simulink model "tm_func"  (R2026a)
settings: Solver=VariableStepAuto  StopTime=100
values from neighbouring files (symbols this model uses):
  q0 = (1 + a - 2*pd) / b    [questao6.m]
  q1 = (pd^2 - a) / b    [questao6.m]
  Tc_perturbacao = 1    [tarefa1.m]
  V_manipulada = 20    [tarefa1.m]
settings Model: Creator=arthu  LastModifiedBy=arthu

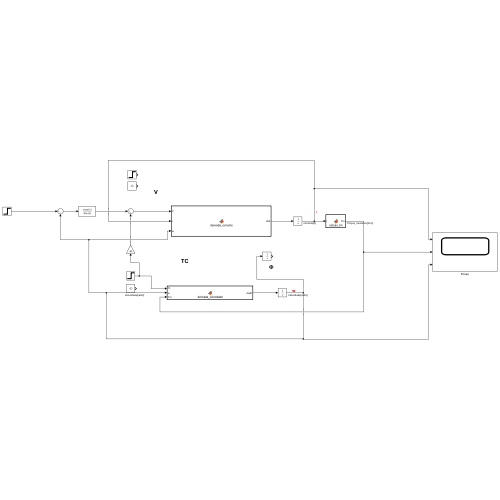
[thumbnail: Simulink's stored preview of the top-level diagram]
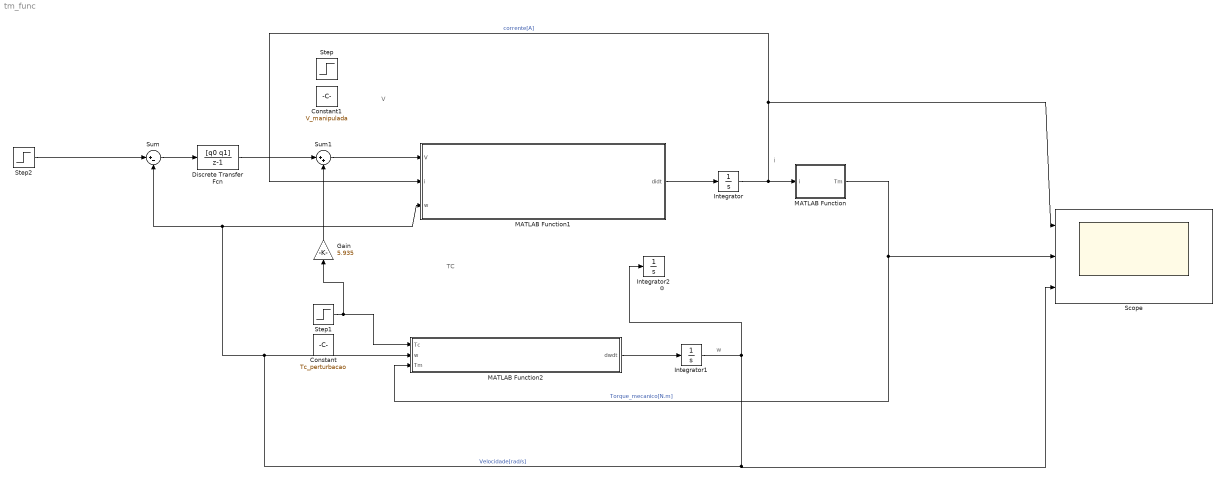
== system tm_func ==
  note: TC
  note: w
  note: i
  note: V
  note: Φ
  Constant : Constant  Value=Tc_perturbacao
  Constant1 : Constant  Value=V_manipulada
  Discrete Transfer Fcn : DiscreteTransferFcn  Numerator=[q0 q1]  Denominator=[1 -1]
  Gain : Gain  Gain=5.935
  Integrator : Integrator
  Integrator1 : Integrator
  Integrator2 : Integrator
  MATLAB Function : MATLAB Function  TreatAsAtomicUnit=on
  MATLAB Function1 : MATLAB Function  TreatAsAtomicUnit=on
  MATLAB Function2 : MATLAB Function  TreatAsAtomicUnit=on
  Scope : Scope  NumInputPorts=3
      settings: ActiveDisplayYMinimum=-11.848227456603485  ActiveDisplayYMaximum=62.852483390197342
  Step : Step  Time=50  InitialValue=20  FinalValue=21  SampleTime=0
  Step1 : Step  Time=50  InitialValue=1  FinalValue=1.1  SampleTime=0
  Step2 : Step  Time=0  FinalValue=25.8  SampleTime=0
  Sum : Sum  Inputs=|+-
  Sum1 : Sum  Inputs=|++
  wires:
  MATLAB Function1/1(didt) -> Integrator/1
  Integrator/1 -> Scope/1, MATLAB Function1/2(i), MATLAB Function/1(i)  "corrente[A]"
  MATLAB Function2/1(dwdt) -> Integrator1/1
  Integrator1/1 -> Scope/3, MATLAB Function2/2(w), Sum/2, MATLAB Function1/3(w), Integrator2/1  "Velocidade[rad/s]"
  MATLAB Function/1(Tm) -> Scope/2, MATLAB Function2/3(Tm)  "Torque_mecanico[N.m]"
  Step1/1 -> Gain/1, MATLAB Function2/1(Tc)
  Step2/1 -> Sum/1
  Sum/1 -> Discrete Transfer Fcn/1
  Gain/1 -> Sum1/2
  Discrete Transfer Fcn/1 -> Sum1/1
  Sum1/1 -> MATLAB Function1/1(V)

== matlab function tm_func/MATLAB Function ==
  data: i input; Tm output
    function Tm = calculo_tm(i)
        % Calculo nao-linear do torque
        if i >= 0
            Tm = 5.26 * (1 - exp(-i));
        else
            Tm = -5.26 * (1 - exp(i));
        end
    end

== matlab function tm_func/MATLAB Function2 ==
  data: Tc input; dwdt output; w input; Tm input
function dwdt = derivada_velocidade(Tc, w, Tm)
% Declarando os parametros locais
B = 0.1;
J = 1;

% EDO Mecanica
dwdt = (Tm - Tc - B*w)/J;
end

== matlab function tm_func/MATLAB Function1 ==
  data: V input; didt output; i input; w input

function didt = derivada_corrente(V, i, w)
% Declarando os parametros locais
R = 10;
L = 0.5;
Km = 1/3;

% EDO Eletrica
didt = (V - R*i - Km*w)/L;
end
